simulink model "Demo_veDYNA_cs"  (Simulink 7.6)
settings: Solver=ode1  SolverMode=SingleTasking  StartTime=0  StopTime=15  FixedStep=1/500  RelTol=1e-3
PreLoadFcn:
  | PreScanveDYNAPreLoadFcn(bdroot);
  | check_NUTS_defined;
  | 
  | assignin('base',['model_closed_' bdroot],false);
PostLoadFcn:
  | PreScanveDYNAPostLoadFcn(bdroot);
  | 
InitFcn:
  | vdy_SetExternalInputSource('ManLongCtrl',1,'Brake','other');
  | vdy_SetExternalInputSource('ManLongCtrl',1,'EngineTorque','other');
  | vdy_SetExternalInputSource('ManLatCtrl',1,'Steering','other');
  | 
  | PreScanveDYNAInitFcn(bdroot);
  | PreScanExperimentInitFcn(bdroot)
StopFcn:
  | PreScanExperimentStopFcn(bdroot)
undefined symbols (not defined in the file): at_period, CPT, DiscIntNeverNeededParam, vm_at_pulsewidth, vm_driver_dflt_gain, x_ini_VRML, y_ini_VRML, z_ini_VRML
libraries: dyna_cpt_lib x93, PreScanSimulinkLibrary x10, PreScanUsefulBlocks x4, simulink x4, anilib x3, dyna_lib x3, simulink_extras x2, dyna_manctrl_lib x2, dyna_road_lib x2, dyna_io_lib x1, dyna_demo_lib x1, dyna_usr_maneuver_states_lib x1
(part 8 of 8)

== system Demo_veDYNA_cs/Vedyna_Vehicle/CPT_MDL/MDL_SW/Wheel/System Instance 7/HCI [1,..,n] ==
  Switch : Constant  Value=CPT.MDL_SW.Wheel{7}.HCI.Switch.v
  Terminator : Terminator
  tag scope: Wheel_7_HCI_SW=global
  wires:
  Switch/1 -> [Wheel_7_HCI_SW]
  [Wheel_7_HCI_SW] -> Terminator/1

== system Demo_veDYNA_cs/Vedyna_Vehicle/CPT_MDL/MDL_SW/Wheel/System Instance 7/pbrm [1,..,4] ==
  Switch : Constant  Value=CPT.MDL_SW.Wheel{7}.pbrm.Switch.v
  Terminator : Terminator
  tag scope: Wheel_7_pbrm_SW=global
  wires:
  Switch/1 -> [Wheel_7_pbrm_SW]
  [Wheel_7_pbrm_SW] -> Terminator/1

== system Demo_veDYNA_cs/Vedyna_Vehicle/CPT_MDL/MDL_SW/Wheel/System Instance 8/HCI [1,..,n] ==
  Switch : Constant  Value=CPT.MDL_SW.Wheel{8}.HCI.Switch.v
  Terminator : Terminator
  tag scope: Wheel_8_HCI_SW=global
  wires:
  Switch/1 -> [Wheel_8_HCI_SW]
  [Wheel_8_HCI_SW] -> Terminator/1

== system Demo_veDYNA_cs/Vedyna_Vehicle/CPT_MDL/MDL_SW/Wheel/System Instance 8/pbrm [1,..,4] ==
  Switch : Constant  Value=CPT.MDL_SW.Wheel{8}.pbrm.Switch.v
  Terminator : Terminator
  tag scope: Wheel_8_pbrm_SW=global
  wires:
  Switch/1 -> [Wheel_8_pbrm_SW]
  [Wheel_8_pbrm_SW] -> Terminator/1

== system Demo_veDYNA_cs/Vedyna_Vehicle/vdy_mdl/Vehicle System/veDYNA Vehicle Subsystem/Brake System/Configurable Subsystem ==
  Brake Pedal Position : Inport
  I/O Vector : Inport  Port=2
  SyncIn : Inport  Port=3
  HCI Switch : Inport  Port=4
  veDYNA Brake Hydraulics : dyna_brakehydraulics_lib/veDYNA Brake Hydraulics  Tag=vedynaBrkHydMask  local_comp_inst=1  system_comp_inst=1
  SyncOut : Outport
  BrkHyd Info : Outport  Port=2
  Master Cylinder Pressure : Outport  Port=3
  Wheel 1 Cylinder Pressure : Outport  Port=4
  Wheel 2 Cylinder Pressure : Outport  Port=5
  Wheel 3 Cylinder Pressure : Outport  Port=6
  Wheel 4 Cylinder Pressure : Outport  Port=7
  Wheel 5 Cylinder Pressure : Outport  Port=8
  Wheel 6 Cylinder Pressure : Outport  Port=9
  Wheel 7 Cylinder Pressure : Outport  Port=10
  Wheel 8 Cylinder Pressure : Outport  Port=11
  wires:
  veDYNA Brake Hydraulics/11 -> Wheel 8 Cylinder Pressure/1
  veDYNA Brake Hydraulics/10 -> Wheel 7 Cylinder Pressure/1
  veDYNA Brake Hydraulics/9 -> Wheel 6 Cylinder Pressure/1
  veDYNA Brake Hydraulics/8 -> Wheel 5 Cylinder Pressure/1
  veDYNA Brake Hydraulics/7 -> Wheel 4 Cylinder Pressure/1
  veDYNA Brake Hydraulics/6 -> Wheel 3 Cylinder Pressure/1
  veDYNA Brake Hydraulics/5 -> Wheel 2 Cylinder Pressure/1
  veDYNA Brake Hydraulics/4 -> Wheel 1 Cylinder Pressure/1
  veDYNA Brake Hydraulics/3 -> Master Cylinder Pressure/1
  veDYNA Brake Hydraulics/2 -> BrkHyd Info/1
  veDYNA Brake Hydraulics/1 -> SyncOut/1
  HCI Switch/1 -> veDYNA Brake Hydraulics/4
  SyncIn/1 -> veDYNA Brake Hydraulics/3
  I/O Vector/1 -> veDYNA Brake Hydraulics/2
  Brake Pedal Position/1 -> veDYNA Brake Hydraulics/1

== system Demo_veDYNA_cs/Vedyna_Vehicle/vdy_mdl/Vehicle System/veDYNA Vehicle Subsystem/Brake System/HCI Switch ==
  SW_BrkHyd_1_HCI : dyna_cpt_lib/CPT_MDL_HCI_SW_ACCESS  Tag=vedynaCPT_MDL_HCI_SW_ACCESS  component=BrkHyd  system_inst=1  parameter=HCI
  HCI Switch : Outport
  wires:
  SW_BrkHyd_1_HCI/1 -> HCI Switch/1

== system Demo_veDYNA_cs/Vedyna_Vehicle/vdy_mdl/Vehicle System/veDYNA Vehicle Subsystem/External Vehicle Inputs (from I/O)/Inputs from I/O ==
  I/O Vector : Inport
  Demux1 : Demux  Outputs=[1,1,1,1]
  ASR Flag : Outport
  ASR Torque : Outport  Port=2
  MSR Flag : Outport  Port=3
  MSR Torque : Outport  Port=4
  wires:
  I/O Vector/1 -> Demux1/1
  Demux1/1 -> ASR Flag/1
  Demux1/2 -> ASR Torque/1
  Demux1/3 -> MSR Flag/1
  Demux1/4 -> MSR Torque/1

== system Demo_veDYNA_cs/Vedyna_Vehicle/vdy_mdl/Vehicle System/veDYNA Vehicle Subsystem/External Vehicle Inputs (from I/O)/Inputs from Maneuver ==
  Maneuver Commands : Inport
  Demux1 : Demux  Outputs=[1,1,1,1,1,1,1,1,1]
  Road mue Wheel 1 : Outport
  Road mue Wheel 2 : Outport  Port=2
  Road mue Wheel 3 : Outport  Port=3
  Road mue Wheel 4 : Outport  Port=4
  Road mue Wheel 5 : Outport  Port=5
  Road mue Wheel 6 : Outport  Port=6
  Hydropulse Flag : Outport  Port=7
  Hydropulse Left (Wheels 1,3,5) : Outport  Port=8
  Hydropulse Right (Wheels 2,4,6) : Outport  Port=9
  wires:
  Demux1/1 -> Road mue Wheel 1/1
  Demux1/2 -> Road mue Wheel 2/1
  Demux1/3 -> Road mue Wheel 3/1
  Demux1/4 -> Road mue Wheel 4/1
  Demux1/5 -> Road mue Wheel 5/1
  Demux1/6 -> Road mue Wheel 6/1
  Demux1/7 -> Hydropulse Flag/1
  Demux1/8 -> Hydropulse Left (Wheels 1,3,5)/1
  Demux1/9 -> Hydropulse Right (Wheels 2,4,6)/1
  Maneuver Commands/1 -> Demux1/1
